simulink model "SLA_1a"  (R2023a)
settings: Solver=ode4  StartTime=0.0  StopTime=20  FixedStep=0.005  RelTol=1e-3
InitFcn:
  | SLA
values from neighbouring files (symbols this model uses):
  K_scheduled = zeros(length(V_op), 2)    [CAL3.m]    (also in CUB.m; DLC2.m; MUS.m; OHZ.m)
  V_op = 5:5:85    [CAL3.m]    (also in CUB.m; DLC2.m; MUS.m; OHZ.m)
  X_track = [linspace(0, runway_length, 200)'; runway_length + R_track * cos(theta_circ(2:end))]    [CAL3.m]    (also in CUB.m = [0; 5000]; DLC2.m = 0:0.1:total_track_length; MUS.m = [0; 2000]; OHZ.m = [0; 2000])
  Y_track = [zeros(200, 1); R_track + R_track * sin(theta_circ(2:end))]    [CAL3.m]    (also in CUB.m = [0; 0]; DLC2.m = zeros(size(X_track)); MUS.m = [0; 0]; OHZ.m = [0; 0])
libraries: simulink x2, slpidlib x1
(part 1 of 2)
settings Model: NumberOfSteps=1000  SnapshotBufferSize=1000  SnapshotInterval=1000  Creator=KBISWAS  LastModifiedBy=KBISWAS

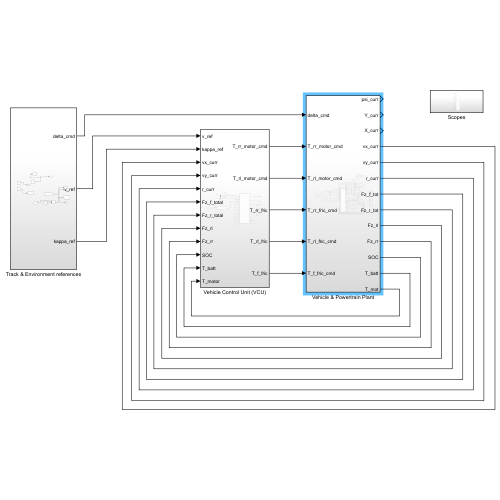
[thumbnail: Simulink's stored preview of the top-level diagram]
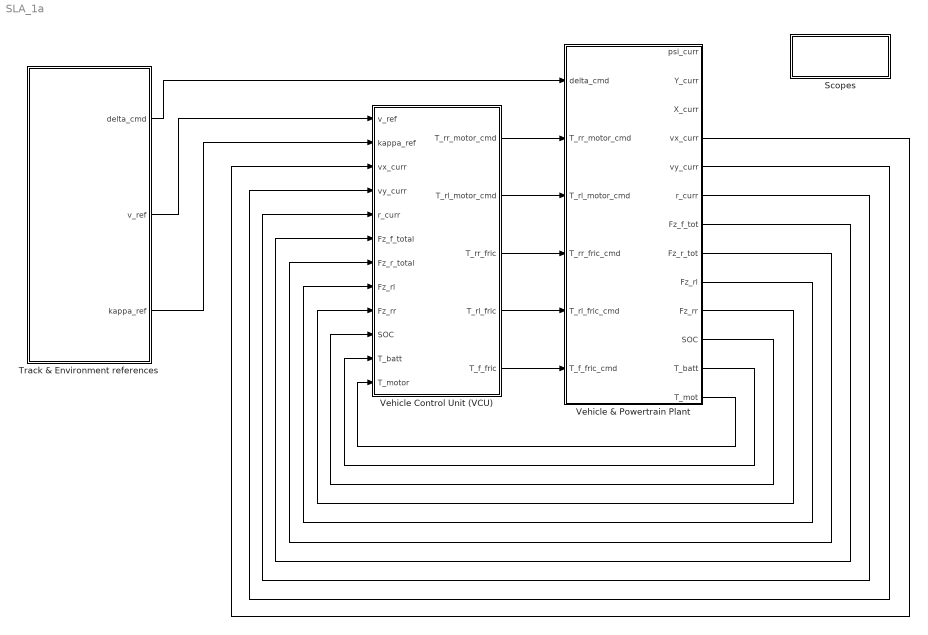
== system SLA_1a ==
  Scopes : Subsystem
  Track & Environment references : Subsystem
  Vehicle & Powertrain Plant : Subsystem
  Vehicle Control Unit (VCU) : Subsystem
  wires:
  Track & Environment references/2(v_ref) -> Vehicle Control Unit (VCU)/1(v_ref)
  Vehicle Control Unit (VCU)/1(T_rr_motor_cmd) -> Vehicle & Powertrain Plant/2(T_rr_motor_cmd)
  Track & Environment references/3(kappa_ref) -> Vehicle Control Unit (VCU)/2(kappa_ref)
  Track & Environment references/1(delta_cmd) -> Vehicle & Powertrain Plant/1(delta_cmd)
  Vehicle Control Unit (VCU)/2(T_rl_motor_cmd) -> Vehicle & Powertrain Plant/3(T_rl_motor_cmd)
  Vehicle Control Unit (VCU)/3(T_rr_fric) -> Vehicle & Powertrain Plant/4(T_rr_fric_cmd)
  Vehicle Control Unit (VCU)/4(T_rl_fric) -> Vehicle & Powertrain Plant/5(T_rl_fric_cmd)
  Vehicle Control Unit (VCU)/5(T_f_fric) -> Vehicle & Powertrain Plant/6(T_f_fric_cmd)
  Vehicle & Powertrain Plant/4(vx_curr) -> Vehicle Control Unit (VCU)/3(vx_curr)
  Vehicle & Powertrain Plant/5(vy_curr) -> Vehicle Control Unit (VCU)/4(vy_curr)
  Vehicle & Powertrain Plant/6(r_curr) -> Vehicle Control Unit (VCU)/5(r_curr)
  Vehicle & Powertrain Plant/7(Fz_f_tot) -> Vehicle Control Unit (VCU)/6(Fz_f_total)
  Vehicle & Powertrain Plant/8(Fz_r_tot) -> Vehicle Control Unit (VCU)/7(Fz_r_total)
  Vehicle & Powertrain Plant/9(Fz_rl) -> Vehicle Control Unit (VCU)/8(Fz_rl)
  Vehicle & Powertrain Plant/10(Fz_rr) -> Vehicle Control Unit (VCU)/9(Fz_rr)
  Vehicle & Powertrain Plant/11(SOC) -> Vehicle Control Unit (VCU)/10(SOC)
  Vehicle & Powertrain Plant/12(T_batt) -> Vehicle Control Unit (VCU)/11(T_batt)
  Vehicle & Powertrain Plant/13(T_mot) -> Vehicle Control Unit (VCU)/12(T_motor)

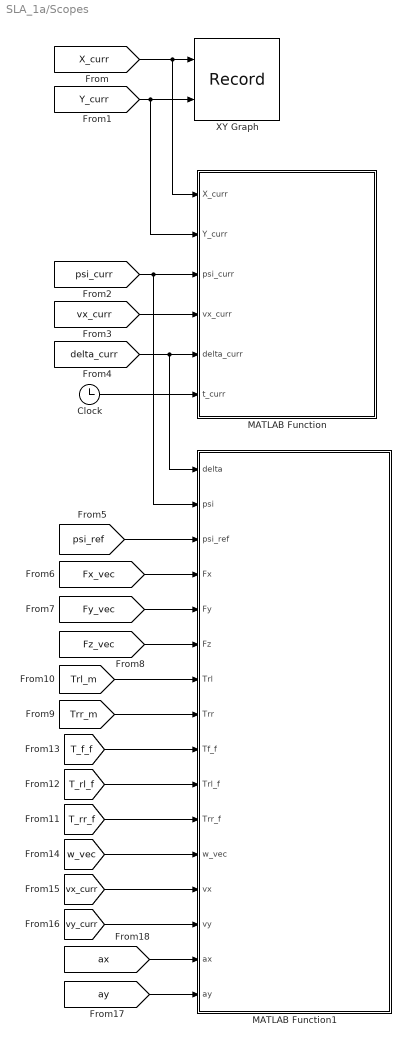
== system SLA_1a/Scopes ==
  Clock : Clock
  MATLAB Function : MATLAB Function  TreatAsAtomicUnit=on
  MATLAB Function1 : MATLAB Function  TreatAsAtomicUnit=on
  XY Graph : Record  FileSettingsInternal="{\"entries\":[{\"content\":{\"excelSettings\":{\"content\":{},\"type\":\"Streamout.ExcelSettings\"}},\"type\":\"Streamout.FileSettingStorage\",\"uuid\":\"\"}],\"packageUris\":[\"http:\\/\\/schema.mathworks.com\\/mf0\\/streamout_blocks\\/R2020a\"],\"version\":\"1.0\"}"  Layout=[1 1]  SignalsInternal="{\"entries\":[{\"content\":{\"signals\":[{\"content\":{\"blockPath\":[],\"dimensions\":[1],\"domain\":\"\",\"lineColor\":\"#a2142f\",\"plots\":[1],\"port\":1,\"signalID\":11566,\"signalName\":\"From\"},\"type\":\"RecordBlkView.Signal\",\"uuid\":\"\"},{\"content\":{\"blockPath\":[],\"dimensions\":[1],\"domain\":\"\",\"lineColor\":\"#139fff\",\"plots\":[1],\"port\":2,\"signalID\":11569,\"signalName\":\"From1\"},\"type\":\"RecordBlkView.Signal\",\"uuid\":\"\"}]},\"type\":\"RecordBlkView.InputSignals\",\"uuid\":\"\"}],\"packageUris\":[\"http:\\/\\/schema.mathworks.com\\/mf0\\/streamout_blocks\\/R2020a\"],\"version\":\"1.0\"}"  VisualizationBindings="{\"xyplotplugin\":{\"info\":[{\"series\":[{\"bindingParametersList\":[{\"parameter\":\"X-Axis\",\"signalID\":11566,\"signalName\":\"From\"},{\"parameter\":\"Y-Axis\",\"signalID\":11569,\"signalName\":\"From1\"}],\"seriesID\":14015}],\"subplotID\":1}]}}"  CompatibilityTag=XY
  wires:
  [X_curr] -> MATLAB Function/1(X_curr), XY Graph/1
  [Y_curr] -> MATLAB Function/2(Y_curr), XY Graph/2
  [psi_curr] -> MATLAB Function/3(psi_curr), MATLAB Function1/2(psi)
  [vx_curr] -> MATLAB Function/4(vx_curr)
  [delta_curr] -> MATLAB Function1/1(delta), MATLAB Function/5(delta_curr)
  Clock/1 -> MATLAB Function/6(t_curr)
  [psi_ref] -> MATLAB Function1/3(psi_ref)
  [Fx_vec] -> MATLAB Function1/4(Fx)
  [Fy_vec] -> MATLAB Function1/5(Fy)
  [Fz_vec] -> MATLAB Function1/6(Fz)
  [Trr_m] -> MATLAB Function1/8(Trr)
  [Trl_m] -> MATLAB Function1/7(Trl)
  [T_f_f] -> MATLAB Function1/9(Tf_f)
  [T_rr_f] -> MATLAB Function1/11(Trr_f)
  [T_rl_f] -> MATLAB Function1/10(Trl_f)
  [w_vec] -> MATLAB Function1/12(w_vec)
  [vx_curr] -> MATLAB Function1/13(vx)
  [vy_curr] -> MATLAB Function1/14(vy)
  [ax] -> MATLAB Function1/15(ax)
  [ay] -> MATLAB Function1/16(ay)

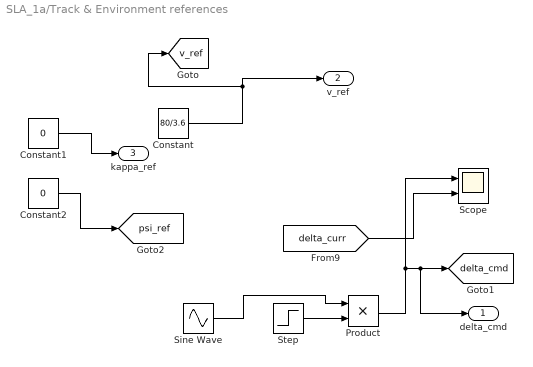
== system SLA_1a/Track & Environment references ==
  Constant : Constant  Value=80/3.6
  Constant1 : Constant  Value=0
  Constant2 : Constant  Value=0
  Product : Product
  Scope : Scope  NumInputPorts=2
  Sine Wave : Sin  Amplitude=0.1  Frequency=4  Phase=0.703  SampleTime=0
  Step : Step  Time=7  SampleTime=0
  delta_cmd : Outport
  v_ref : Outport  Port=2
  kappa_ref : Outport  Port=3
  tag scope: delta_cmd=global, psi_ref=global, v_ref=global
  wires:
  Constant2/1 -> [psi_ref]
  Constant1/1 -> kappa_ref/1
  Constant/1 -> v_ref/1, [v_ref]
  Product/1 -> [delta_cmd], delta_cmd/1, Scope/1
  [delta_curr] -> Scope/2
  Step/1 -> Product/2
  Sine Wave/1 -> Product/1

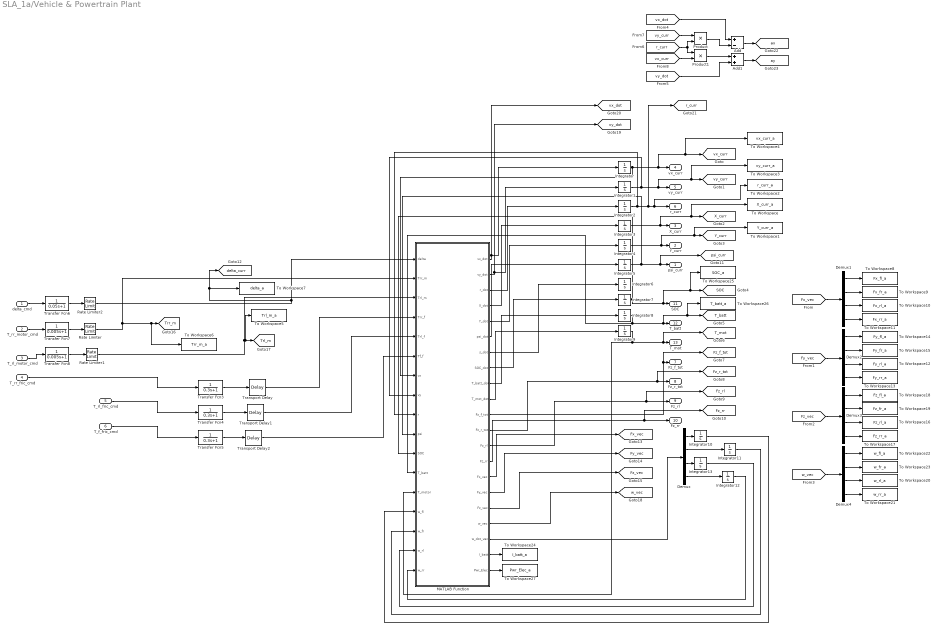
== system SLA_1a/Vehicle & Powertrain Plant ==
  delta_cmd : Inport
  T_rr_motor_cmd : Inport  Port=2
  T_rl_motor_cmd : Inport  Port=3
  T_rr_fric_cmd : Inport  Port=4
  T_rl_fric_cmd : Inport  Port=5
  T_f_fric_cmd : Inport  Port=6
  Add : Sum  Inputs=+-
  Add1 : Sum
  Demux{,1..4} (5 alike) : Demux
  Integrator : Integrator  InitialCondition=5
  Integrator{1..6,10..13} (10 alike) : Integrator
  Integrator7 : Integrator  InitialCondition=0.9
  Integrator8 : Integrator  InitialCondition=30
  Integrator9 : Integrator  InitialCondition=30
  MATLAB Function : MATLAB Function  TreatAsAtomicUnit=on
  Product : Product
  Product1 : Product
  Rate Limiter : RateLimiter  RisingSlewLimit=500  FallingSlewLimit=-500  SampleTimeMode=inherited
  Rate Limiter1 : RateLimiter  RisingSlewLimit=500  FallingSlewLimit=-500  SampleTimeMode=inherited
  Rate Limiter2 : RateLimiter  RisingSlewLimit=10  FallingSlewLimit=-10  SampleTimeMode=inherited
  To Workspace : ToWorkspace  VariableName=X_curr_a  SaveFormat=Timeseries  SampleTime=-1
  To Workspace1 : ToWorkspace  VariableName=Y_curr_a  SaveFormat=Timeseries  SampleTime=-1
  To Workspace10 : ToWorkspace  VariableName=Fx_rl_a  SaveFormat=Timeseries  SampleTime=-1
  To Workspace11 : ToWorkspace  VariableName=Fx_rr_a  SaveFormat=Timeseries  SampleTime=-1
  To Workspace12 : ToWorkspace  VariableName=Fy_rl_a  SaveFormat=Timeseries  SampleTime=-1
  To Workspace13 : ToWorkspace  VariableName=Fy_rr_a  SaveFormat=Timeseries  SampleTime=-1
  To Workspace14 : ToWorkspace  VariableName=Fy_fl_a  SaveFormat=Timeseries  SampleTime=-1
  To Workspace15 : ToWorkspace  VariableName=Fy_fr_a  SaveFormat=Timeseries  SampleTime=-1
  To Workspace16 : ToWorkspace  VariableName=Fz_rl_a  SaveFormat=Timeseries  SampleTime=-1
  To Workspace17 : ToWorkspace  VariableName=Fz_rr_a  SaveFormat=Timeseries  SampleTime=-1
  To Workspace18 : ToWorkspace  VariableName=Fz_fl_a  SaveFormat=Timeseries  SampleTime=-1
  To Workspace19 : ToWorkspace  VariableName=Fz_fr_a  SaveFormat=Timeseries  SampleTime=-1
  To Workspace2 : ToWorkspace  VariableName=r_curr_a  SaveFormat=Timeseries  SampleTime=-1
  To Workspace20 : ToWorkspace  VariableName=w_rl_a  SaveFormat=Timeseries  SampleTime=-1
  To Workspace21 : ToWorkspace  VariableName=w_rr_a  SaveFormat=Timeseries  SampleTime=-1
  To Workspace22 : ToWorkspace  VariableName=w_fl_a  SaveFormat=Timeseries  SampleTime=-1
  To Workspace23 : ToWorkspace  VariableName=w_fr_a  SaveFormat=Timeseries  SampleTime=-1
  To Workspace24 : ToWorkspace  VariableName=I_batt_a  SaveFormat=Timeseries  SampleTime=-1
  To Workspace25 : ToWorkspace  VariableName=SOC_a  SaveFormat=Timeseries  SampleTime=-1
  To Workspace26 : ToWorkspace  VariableName=T_batt_a  SaveFormat=Timeseries  SampleTime=-1
  To Workspace27 : ToWorkspace  VariableName=Pwr_Elec_a  SaveFormat=Timeseries  SampleTime=-1
  To Workspace3 : ToWorkspace  VariableName=vy_curr_a  SaveFormat=Timeseries  SampleTime=-1
  To Workspace4 : ToWorkspace  VariableName=vx_curr_a  SaveFormat=Timeseries  SampleTime=-1
  To Workspace5 : ToWorkspace  VariableName=Trl_m_a  SaveFormat=Timeseries  SampleTime=-1
  To Workspace6 : ToWorkspace  VariableName=Trr_m_a  SaveFormat=Timeseries  SampleTime=-1
  To Workspace7 : ToWorkspace  VariableName=delta_a  SaveFormat=Timeseries  SampleTime=-1
  To Workspace8 : ToWorkspace  VariableName=Fx_fl_a  SaveFormat=Timeseries  SampleTime=-1
  To Workspace9 : ToWorkspace  VariableName=Fx_fr_a  SaveFormat=Timeseries  SampleTime=-1
  Transfer Fcn3 : TransferFcn  Denominator=[0.3 1]
  Transfer Fcn4 : TransferFcn  Denominator=[0.3 1]
  Transfer Fcn5 : TransferFcn  Denominator=[0.3 1]
  Transfer Fcn6 : TransferFcn  Numerator=1  Denominator=[0.05 1]
  Transfer Fcn7 : TransferFcn  Denominator=[0.005 1]
  Transfer Fcn8 : TransferFcn  Denominator=[0.005 1]
  Transport Delay : TransportDelay  DelayTime=0.03
  Transport Delay1 : TransportDelay  DelayTime=0.03
  Transport Delay2 : TransportDelay  DelayTime=0.03
  psi_curr : Outport
  Y_curr : Outport  Port=2
  X_curr : Outport  Port=3
  vx_curr : Outport  Port=4
  vy_curr : Outport  Port=5
  r_curr : Outport  Port=6
  Fz_f_tot : Outport  Port=7
  Fz_r_tot : Outport  Port=8
  Fz_rl : Outport  Port=9
  Fz_rr : Outport  Port=10
  SOC : Outport  Port=11
  T_batt : Outport  Port=12
  T_mot : Outport  Port=13
  tag scope: Fx_vec=global, Fy_vec=global, Fz_f_tot=global, Fz_r_tot=global, Fz_rl=global, Fz_rr=global, Fz_vec=global, SOC=global, T_batt=global, T_mot=global, Trl_m=global, Trr_m=global, X_curr=global, Y_curr=global, ax=global, ay=global, delta_curr=global, psi_curr=global, r_curr=global, vx_curr=global, vx_dot=global, vy_curr=global, vy_dot=global, w_vec=global
  wires:
  delta_cmd/1 -> Transfer Fcn6/1
  T_rr_fric_cmd/1 -> Transfer Fcn3/1
  T_rl_fric_cmd/1 -> Transfer Fcn4/1
  T_f_fric_cmd/1 -> Transfer Fcn5/1
  Transfer Fcn6/1 -> Rate Limiter2/1
  Rate Limiter/1 -> MATLAB Function/2(Trr_m), To Workspace6/1, [Trr_m]
  Rate Limiter1/1 -> MATLAB Function/3(Trl_m), To Workspace5/1, [Trl_m]
  Transfer Fcn3/1 -> Transport Delay/1
  Transfer Fcn4/1 -> Transport Delay1/1
  Transfer Fcn5/1 -> Transport Delay2/1
  MATLAB Function/1(vx_dot) -> [vx_dot], Integrator/1
  MATLAB Function/2(vy_dot) -> [vy_dot], Integrator1/1
  MATLAB Function/3(r_dot) -> Integrator2/1
  MATLAB Function/4(X_dot) -> Integrator3/1
  MATLAB Function/5(Y_dot) -> Integrator4/1
  MATLAB Function/6(psi_dot) -> Integrator5/1
  MATLAB Function/7(s_dot) -> Integrator6/1
  MATLAB Function/8(SOC_dot) -> Integrator7/1
  Integrator/1 -> MATLAB Function/7(vx), To Workspace4/1, [vx_curr], vx_curr/1
  Integrator1/1 -> MATLAB Function/8(vy), To Workspace3/1, [vy_curr], vy_curr/1
  Integrator2/1 -> [r_curr], To Workspace2/1, r_curr/1, MATLAB Function/9(r)
  Integrator5/1 -> MATLAB Function/10(psi), [psi_curr], psi_curr/1
  Integrator8/1 -> MATLAB Function/12(T_batt), To Workspace26/1, [T_batt], T_batt/1
  Integrator9/1 -> MATLAB Function/13(T_motor), [T_mot], T_mot/1
  Integrator4/1 -> To Workspace1/1, [Y_curr], Y_curr/1
  Integrator3/1 -> To Workspace/1, [X_curr], X_curr/1
  MATLAB Function/11(Fz_f_tot) -> [Fz_f_tot], Fz_f_tot/1
  Integrator7/1 -> MATLAB Function/11(SOC), To Workspace25/1, [SOC], SOC/1
  MATLAB Function/14(Fz_rr) -> [Fz_rr], Fz_rr/1
  MATLAB Function/15(Fx_vec) -> [Fx_vec]
  MATLAB Function/17(Fz_vec) -> [Fz_vec]
  MATLAB Function/9(T_batt_dot) -> Integrator8/1
  MATLAB Function/10(T_mot_dot) -> Integrator9/1
  MATLAB Function/12(Fz_r_tot) -> [Fz_r_tot], Fz_r_tot/1
  MATLAB Function/13(Fz_rl) -> [Fz_rl], Fz_rl/1
  MATLAB Function/16(Fy_vec) -> [Fy_vec]
  MATLAB Function/18(w_vec) -> [w_vec]
  Demux/4 -> Integrator12/1
  Demux/3 -> Integrator13/1
  Demux/2 -> Integrator11/1
  Demux/1 -> Integrator10/1
  MATLAB Function/19(w_dot_vec) -> Demux/1
  Integrator10/1 -> MATLAB Function/14(w_fl)
  Integrator11/1 -> MATLAB Function/15(w_fr)
  Integrator12/1 -> MATLAB Function/17(w_rr)
  Integrator13/1 -> MATLAB Function/16(w_rl)
  T_rr_motor_cmd/1 -> Transfer Fcn7/1
  Transfer Fcn7/1 -> Rate Limiter/1
  Transfer Fcn8/1 -> Rate Limiter1/1
  T_rl_motor_cmd/1 -> Transfer Fcn8/1
  [Fx_vec] -> Demux1/1
  Demux1/1 -> To Workspace8/1
  Demux1/2 -> To Workspace9/1
  Demux1/3 -> To Workspace10/1
  Demux1/4 -> To Workspace11/1
  Demux2/2 -> To Workspace15/1
  Demux2/4 -> To Workspace13/1
  Demux2/1 -> To Workspace14/1
  [Fy_vec] -> Demux2/1
  Demux2/3 -> To Workspace12/1
  [Fz_vec] -> Demux3/1
  Demux3/1 -> To Workspace18/1
  Demux3/3 -> To Workspace16/1
  Demux3/4 -> To Workspace17/1
  Demux3/2 -> To Workspace19/1
  Demux4/2 -> To Workspace23/1
  Demux4/4 -> To Workspace21/1
  Demux4/1 -> To Workspace22/1
  Demux4/3 -> To Workspace20/1
  [w_vec] -> Demux4/1
  [vy_curr] -> Product/1
  [r_curr] -> Product1/1, Product/2
  Product/1 -> Add/2
  [vx_dot] -> Add/1
  [vx_curr] -> Product1/2
  Product1/1 -> Add1/1
  [vy_dot] -> Add1/2
  Add/1 -> [ax]
  Add1/1 -> [ay]
  MATLAB Function/20(I_batt) -> To Workspace24/1
  MATLAB Function/21(Pwr_Elec) -> To Workspace27/1
  Rate Limiter2/1 -> MATLAB Function/1(delta), To Workspace7/1, [delta_curr]
  Transport Delay/1 -> MATLAB Function/4(Trr_f)
  Transport Delay1/1 -> MATLAB Function/5(Trl_f)
  Transport Delay2/1 -> MATLAB Function/6(Tf_f)

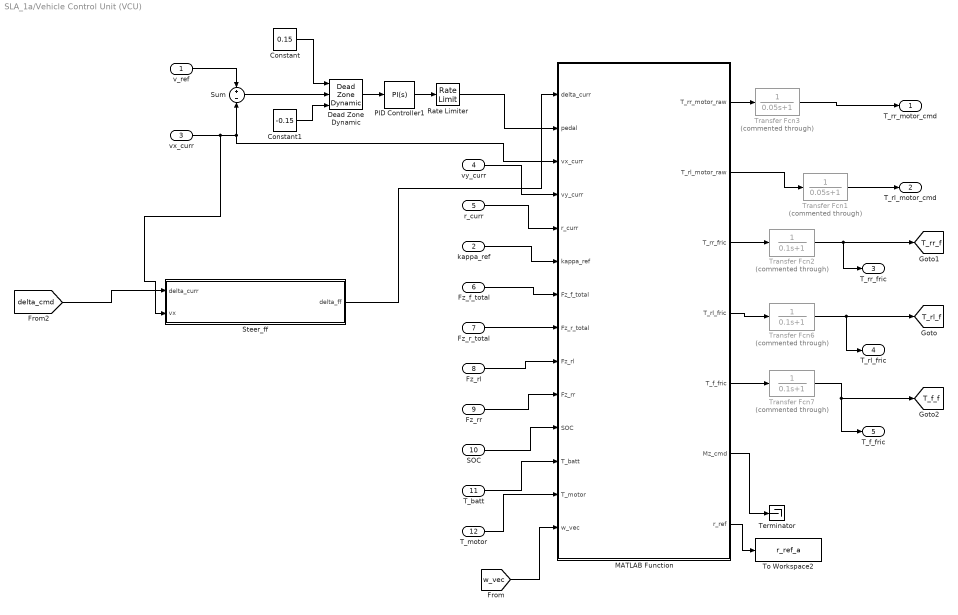
== system SLA_1a/Vehicle Control Unit (VCU) ==
  v_ref : Inport
  kappa_ref : Inport  Port=2
  vx_curr : Inport  Port=3
  vy_curr : Inport  Port=4
  r_curr : Inport  Port=5
  Fz_f_total : Inport  Port=6
  Fz_r_total : Inport  Port=7
  Fz_rl : Inport  Port=8
  Fz_rr : Inport  Port=9
  SOC : Inport  Port=10
  T_batt : Inport  Port=11
  T_motor : Inport  Port=12
  Constant : Constant  Value=0.15
  Constant1 : Constant  Value=-0.15
  Dead Zone Dynamic : simulink/Discontinuities/Dead Zone Dynamic
  MATLAB Function : MATLAB Function  TreatAsAtomicUnit=on
  PID Controller1 : slpidlib/PID Controller  Controller=PI  Form=Parallel  TimeDomain=Continuous-time  UseExternalTs=off  SampleTime=-1  IntegratorMethod=Forward Euler  FilterMethod=Forward Euler  ControllerParametersSource=internal  P=0.2  I=0.1  UseKiTs=off  D=0  N=100  UseFilter=on  TunerSelectOption=Transfer Function Based (PID Tuner App)  InitialConditionSource=internal  InitialConditionForIntegrator=0  InitialConditionForFilter=0  DifferentiatorICPrevScaledInput=0  ExternalReset=none  TrackingMode=off  Kt=1  LimitOutput=on  SatLimitsSource=internal  UpperSaturationLimit=1  LowerSaturationLimit=-1  LinearizeAsGain=on  AntiWindupMode=clamping  Kb=1  LimitIntegrator=off  UpperIntegratorSaturationLimit=inf  LowerIntegratorSaturationLimit=-inf  POutMin=[]  POutMax=[]  IOutMin=[]  IOutMax=[]  DOutMin=[]  DOutMax=[]  NOutMin=[]  NOutMax=[]  SumOutMin=[]  SumOutMax=[]  SaturationOutMin=[]  SaturationOutMax=[]  PParamMin=[]  PParamMax=[]  IParamMin=[]  IParamMax=[]  DParamMin=[]  DParamMax=[]  NParamMin=[]  NParamMax=[]  KbParamMin=[]  KbParamMax=[]  KtParamMin=[]  KtParamMax=[]  KbOutMin=[]  KbOutMax=[]  KtOutMin=[]  KtOutMax=[]  IntegratorOutMin=[]  IntegratorOutMax=[]  FilterOutMin=[]  FilterOutMax=[]  SumI1OutMin=[]  SumI1OutMax=[]  SumI2OutMin=[]  SumI2OutMax=[]  SumI3OutMin=[]  SumI3OutMax=[]  SumI4OutMin=[]  SumI4OutMax=[]  SumDOutMin=[]  SumDOutMax=[]  DifferentiatorOutMin=[]  DifferentiatorOutMax=[]  FilterDiffOutCoefMin=[]  FilterDiffOutCoefMax=[]  ReciprocalOutMin=[]  ReciprocalOutMax=[]  SumDenOutMin=[]  SumDenOutMax=[]  SumNumOutMin=[]  SumNumOutMax=[]  DivideOutMin=[]  DivideOutMax=[]  UdiffTsProdOutMin=[]  UdiffTsProdOutMax=[]  NTsProdOutMin=[]  NTsProdOutMax=[]  UintegralTsProdOutMin=[]  UintegralTsProdOutMax=[]  UngainTsProdOutMin=[]  UngainTsProdOutMax=[]  ClampingZeroOutDataTypeStr=Inherit: Inherit via back propagation  ClampingZeroOutMin=[]  ClampingZeroOutMax=[]  FilterDenConstantOutDataTypeStr=Inherit: Inherit via back propagation  FilterDenConstantOutMin=[]  FilterDenConstantOutMax=[]  PCopyOutDataTypeStr=Inherit: Inherit via back propagation  PCopyOutMin=[]  PCopyOutMax=[]  NCopyOutDataTypeStr=Inherit: Inherit via back propagation  NCopyOutMin=[]  NCopyOutMax=[]  IntegratorContinuousStateAttributes=''  IntegratorStateMustResolveToSignalObject=off  IntegratorRTWStateStorageClass=Auto  FilterContinuousStateAttributes=''  FilterStateMustResolveToSignalObject=off  FilterRTWStateStorageClass=Auto  ParallelPVariant=InternalParameters  IdealPVariant=Disabled  IVariant=InternalParameters  DVariant=Disabled  IntegratorVariant=Continuous  SatVariant=Enabled  AWVariant=ContClampingParallel  PCopyVariant=Disabled  TRVariant=Disabled  FdbkBlocksVariant=Forward  IdealPFdbkVariant=Disabled  SatFdbkVariant=Disabled  DerivativeFilterVariant=Disabled  NVariant=Disabled  NCopyVariant=Disabled_SignalSpec  FilterICVariant=Disabled  IntegratorICVariant=InternalICs  ExternalResetVariant=Disabled  TRSumVariant=Passthrough  SumFdbkVariant=Disabled  SumVariant=Sum_PI  TsampFilterVariant=InternalTs  TsampNgainVariant=Passthrough  TsampIntegralVariant=Disabled_SignalSpec  ExternalSaturationOutDataTypeStr=Inherit: Same as second input
  Rate Limiter : RateLimiter  RisingSlewLimit=2  FallingSlewLimit=-4  SampleTimeMode=inherited
  Steer_ff : Subsystem
  Sum : Sum  Inputs=+-
  Terminator : Terminator
  To Workspace2 : ToWorkspace  VariableName=r_ref_a  SaveFormat=Timeseries  SampleTime=-1
  Transfer Fcn1 : TransferFcn  Commented=through  Denominator=[0.05 1]
  Transfer Fcn2 : TransferFcn  Commented=through  Denominator=[0.1 1]
  Transfer Fcn3 : TransferFcn  Commented=through  Denominator=[0.05 1]
  Transfer Fcn6 : TransferFcn  Commented=through  Denominator=[0.1 1]
  Transfer Fcn7 : TransferFcn  Commented=through  Denominator=[0.1 1]
  T_rr_motor_cmd : Outport
  T_rl_motor_cmd : Outport  Port=2
  T_rr_fric : Outport  Port=3
  T_rl_fric : Outport  Port=4
  T_f_fric : Outport  Port=5
  tag scope: T_f_f=global, T_rl_f=global, T_rr_f=global
  wires:
  v_ref/1 -> Sum/1
  vy_curr/1 -> MATLAB Function/4(vy_curr)
  r_curr/1 -> MATLAB Function/5(r_curr)
  kappa_ref/1 -> MATLAB Function/6(kappa_ref)
  Fz_f_total/1 -> MATLAB Function/7(Fz_f_total)
  Fz_r_total/1 -> MATLAB Function/8(Fz_r_total)
  Fz_rl/1 -> MATLAB Function/9(Fz_rl)
  Fz_rr/1 -> MATLAB Function/10(Fz_rr)
  SOC/1 -> MATLAB Function/11(SOC)
  T_batt/1 -> MATLAB Function/12(T_batt)
  T_motor/1 -> MATLAB Function/13(T_motor)
  Rate Limiter/1 -> MATLAB Function/2(pedal)
  MATLAB Function/1(T_rr_motor_raw) -> Transfer Fcn3/1
  MATLAB Function/2(T_rl_motor_raw) -> Transfer Fcn1/1
  MATLAB Function/3(T_rr_fric) -> Transfer Fcn2/1
  MATLAB Function/4(T_rl_fric) -> Transfer Fcn6/1
  MATLAB Function/5(T_f_fric) -> Transfer Fcn7/1
  MATLAB Function/6(Mz_cmd) -> Terminator/1
  [w_vec] -> MATLAB Function/14(w_vec)
  MATLAB Function/7(r_ref) -> To Workspace2/1
  Steer_ff/1(delta_ff) -> MATLAB Function/1(delta_curr)
  [delta_cmd] -> Steer_ff/1(delta_curr)
  Transfer Fcn3/1 -> T_rr_motor_cmd/1
  Transfer Fcn1/1 -> T_rl_motor_cmd/1
  Transfer Fcn2/1 -> T_rr_fric/1, [T_rr_f]
  Transfer Fcn6/1 -> T_rl_fric/1, [T_rl_f]
  Transfer Fcn7/1 -> T_f_fric/1, [T_f_f]
  Dead Zone Dynamic/1 -> PID Controller1/1
  Constant/1 -> Dead Zone Dynamic/1
  Sum/1 -> Dead Zone Dynamic/2
  PID Controller1/1 -> Rate Limiter/1
  Constant1/1 -> Dead Zone Dynamic/3
  vx_curr/1 -> Steer_ff/2(vx), MATLAB Function/3(vx_curr), Sum/2

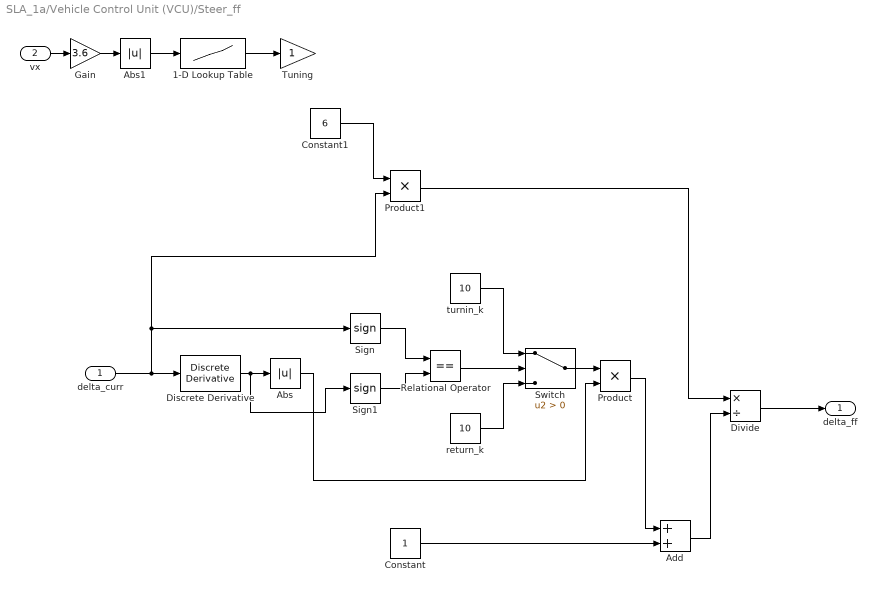
== system SLA_1a/Vehicle Control Unit (VCU)/Steer_ff ==
  delta_curr : Inport
  vx : Inport  Port=2
  1-D Lookup Table : Lookup_n-D  NumberOfTableDimensions=1  LookupTableObject=''  BreakpointsForDimension1=[0 20 40 60 80 100 120 140 160 180 200]  BreakpointsForDimension1FirstPoint=10  BreakpointsForDimension2FirstPoint=10  BreakpointsForDimension1Spacing=12  BreakpointsForDimension2Spacing=12  IndexSearchMethod=Evenly spaced points  Table=[0 2 3.5 3.5 3.5 3.5 3.5 3.5 3 2.5 2]  InterpMethod=Akima spline  DiagnosticForOutOfRangeInput=Error  InternalRulePriority=Speed  RndMeth=Simplest
  Abs : Abs  SaturateOnIntegerOverflow=off
  Abs1 : Abs  SaturateOnIntegerOverflow=off
  Add : Sum
  Constant : Constant
  Constant1 : Constant  Value=6
  Discrete Derivative : simulink/Discrete/Discrete Derivative  gainval=1.0  ICPrevScaledInput=0.0  OutMin=[]  OutMax=[]  OutDataType=fixdt(1, 16)  OutScaling=2^-10  DoSatur=off
  Divide : Product  Inputs=*/
  Gain : Gain  Gain=3.6
  Product : Product
  Product1 : Product
  Relational Operator : RelationalOperator  Operator===  OutDataTypeStr=boolean  RndMeth=Simplest  InputSameDT=off
  Sign : Signum
  Sign1 : Signum
  Switch : Switch  Criteria=u2 > Threshold  SaturateOnIntegerOverflow=off  InputSameDT=off
  Tuning : Gain
  return_k : Constant  Value=10
  turnin_k : Constant  Value=10
  delta_ff : Outport
  wires:
  Product1/1 -> Divide/1
  return_k/1 -> Switch/3
  Switch/1 -> Product/1
  Product/1 -> Add/1
  Sign/1 -> Relational Operator/1
  delta_curr/1 -> Discrete Derivative/1, Product1/2, Sign/1
  Relational Operator/1 -> Switch/2
  Add/1 -> Divide/2
  Discrete Derivative/1 -> Sign1/1, Abs/1
  Abs/1 -> Product/2
  Constant/1 -> Add/2
  Sign1/1 -> Relational Operator/2
  Divide/1 -> delta_ff/1
  turnin_k/1 -> Switch/1
  vx/1 -> Gain/1
  1-D Lookup Table/1 -> Tuning/1
  Gain/1 -> Abs1/1
  Constant1/1 -> Product1/1
  Abs1/1 -> 1-D Lookup Table/1

== matlab function SLA_1a/Scopes/MATLAB Function ==
  settings: updateMethod=DISCRETE
  data: X_curr input; Y_curr input; psi_curr input; vx_curr input; delta_curr input; t_curr input; X_track parameter; Y_track parameter
function live_track_plotter(X_curr, Y_curr, psi_curr, vx_curr, delta_curr, t_curr, X_track, Y_track)
    coder.extrinsic('figure', 'plot', 'hold', 'axis', 'title', 'xlabel', 'ylabel', 'set', 'drawnow', 'animatedline', 'addpoints', 'legend', 'grid', 'patch', 'text');
    
    persistent hFig hCar hTrail hText counter 
    
    if isempty(counter)
        counter = 0;
        
        hFig = figure('Name', 'Circular acceleration tracking', 'Color', 'w', 'Position', [100, 100, 800, 600]);
        plot(X_track, Y_track, '--', 'Color', [0.4 0.4 0.4], 'LineWidth', 1.5); hold on;
        
        plot(X_track(1), Y_track(1), 'ko', 'MarkerSize', 10, 'MarkerFaceColor', 'g', 'LineWidth', 1.5);
        text(X_track(1) - 50, Y_track(1) + 70, 'Start / Finish', 'FontSize', 10, 'FontWeight', 'bold', 'Color', 'k', 'BackgroundColor', [1 1 1 0.7]);
        
        hTrail = animatedline('Color', 'b', 'LineWidth', 1.5);
        
        hCar = patch(0, 0, [0.8 0 0], 'EdgeColor', 'k', 'LineWidth', 1);
        set(hCar, 'FaceAlpha', 0.8); 
        
        hText = text(0, 0, ' Init...', 'FontSize', 10, 'FontWeight', 'bold', 'BackgroundColor', [1 1 1 0.8], 'EdgeColor', 'k', 'Margin', 2);
        
        axis equal; grid on;
        title('Live Vehicle Tracking with Telemetry');
        xlabel('X Position (meters)'); ylabel('Y Position (meters)');
        legend('Reference Track', 'Start/Finish', 'Driven Path', 'EV Position & Heading', 'Telemetry', 'Location', 'best');
    end
    counter = counter + 1;
    
    if mod(counter, 10) == 0
        addpoints(hTrail, X_curr, Y_curr);
        
        % --- REALISTIC 1:1 VEHICLE SCALING ---
        L_vis = 4.5; % 4.5 meters long
        W_vis = 1.9; % 1.9 meters wide
        % ------------------------------------
        
        base_X = [L_vis/2,  L_vis*0.3,   0,       -L_vis*0.35, -L_vis/2,  -L_vis/2,   -L_vis*0.35,  0,        L_vis*0.3,   L_vis/2];
        base_Y = [0,        W_vis*0.45, W_vis/2,  W_vis/2,     W_vis*0.3, -W_vis*0.3, -W_vis/2,    -W_vis/2, -W_vis*0.45, 0];
        
        R = [cos(psi_curr), -sin(psi_curr); 
             sin(psi_curr),  cos(psi_curr)];
             
        rotated_coords = R * [base_X; base_Y];
        final_X = rotated_coords(1, :) + X_curr;
        final_Y = rotated_coords(2, :) + Y_curr;
        
        set(hCar, 'XData', final_X, 'YData', final_Y);
        
        speed_kmh = vx_curr * 3.6;
        steer_deg = delta_curr * (180 / pi);
        
        telemetry_str = sprintf(' Spd: %.1f km/h\n Steer. Ang.: %.1f deg', speed_kmh, steer_deg);
        
        % Brought the text box much closer to the scaled vehicle
        set(hText, 'Position', [X_curr + 10, Y_curr + 10], 'String', telemetry_str);
        
        drawnow limitrate; 
    end
end

== matlab function SLA_1a/Scopes/MATLAB Function1 ==
  settings: updateMethod=DISCRETE
  data: delta input; psi input; psi_ref input; Fx input; Fy input; Fz input; Trl input; Trr input; Tf_f input; Trl_f input; Trr_f input; w_vec input; vx input; vy input; ax input; ay input
function vehicle_frame_plotter(delta, psi, psi_ref, Fx, Fy, Fz, Trl, Trr, Tf_f, Trl_f, Trr_f, w_vec, vx, vy, ax, ay)
    coder.extrinsic('figure', 'plot', 'hold', 'axis', 'title', 'set', 'drawnow', 'patch', 'text', 'line', 'quiver', 'sprintf');
    
    persistent hWheels hSteer hSpokes hPsiRef hPsiAct hFlags hTqFlags hMotors hAxleFront hCircles hGdots hSwLabel hRwLabel hAngleLabel hVelArrow hAccArrow hVelText hAccText hCrosshairs counter
    
    if isempty(counter)
        % =====================================================================
        % STRICT CODER INITIALIZATION
        % =====================================================================
        counter = 0;
        hSteer = 0.0; hPsiRef = 0.0; hPsiAct = 0.0; hAxleFront = 0.0;
        hWheels = zeros(1,4); hFlags = zeros(1,4); hTqFlags = zeros(1,2); hMotors = zeros(1,2);
        hSpokes = zeros(1,3); hCircles = zeros(1,4); hGdots = zeros(1,4);
        hSwLabel = 0.0; hRwLabel = 0.0; hAngleLabel = 0.0;
        hVelArrow = 0.0; hAccArrow = 0.0; hVelText = 0.0; hAccText = 0.0;
        hCrosshairs = zeros(1,2);
        
        figure('Name', 'Vehicle Frame Telemetry - Car A', 'Color', 'w', 'Position', [100, 100, 750, 750]);
        hold on;
        
        % Chassis Outline & Front Axle
        plot([-1, 1, 1, -1, -1], [2, 2, -2, -2, 2], 'k', 'LineWidth', 2);
        hAxleFront = double(line([1, -1], [1.5, 1.5], 'Color', [0.2 0.2 0.2], 'LineWidth', 2));
        
        % Wheels Array Setup [FL, FR, RL, RR]
        for i = 1:4; hWheels(i) = double(patch(0, 0, [0.3 0.3 0.3])); end
        
        % =====================================================================
        % FRICTION CIRCLES, STEERING WHEEL, & YAW VECTORS
        % =====================================================================
        th_c = 0:0.1:2*pi;
        circle_x = cos(th_c); circle_y = sin(th_c);
        c_pos = [-2.0, 2.3; 2.0, 2.3; -2.0, -2.3; 2.0, -2.3]; 
        for i = 1:4
            hCircles(i) = double(plot(c_pos(i,1) + 0.5*circle_x, c_pos(i,2) + 0.5*circle_y, 'Color', [0.6 0 0.6], 'LineStyle', '--', 'LineWidth', 1.2));
            hGdots(i) = double(plot(c_pos(i,1), c_pos(i,2), 'mo', 'MarkerFaceColor', 'm', 'MarkerSize', 5));
        end
        
        hSteer = double(plot(0.4*cos(th_c), 0.4*sin(th_c) + 0.5, 'k', 'LineWidth', 3));
        hSpokes(1) = double(line([0, 0], [0.5, 0.5], 'Color', 'k', 'LineWidth', 2.5));
        hSpokes(2) = double(line([0, 0], [0.5, 0.5], 'Color', 'k', 'LineWidth', 2.5));
        hSpokes(3) = double(line([0, 0], [0.5, 0.5], 'Color', 'k', 'LineWidth', 2.5));
        
        hPsiRef = double(quiver(0, 1.8, 0, 0.8, 'r', 'LineWidth', 2.5, 'MaxHeadSize', 2));
        hPsiAct = double(quiver(0, 1.8, 0, 0.8, 'b', 'LineWidth', 2.5, 'MaxHeadSize', 2));
        
        for i = 1:4; hFlags(i) = double(text(0, 0, '', 'FontSize', 8, 'BackgroundColor', [1 1 1 0.8], 'EdgeColor', 'k')); end
        
        % =====================================================================
        % VEHICLE A POWERTRAIN GRAPHIC (Dual Motors)
        % =====================================================================
        m_b = [-.15, .15, .15, -.15]; m_w = [.2, .2, -.2, -.2];
        hMotors(1) = double(patch(m_b - 0.6, m_w - 1.5, [0.5 0.5 0.5])); % Left Motor
        hMotors(2) = double(patch(m_b + 0.6, m_w - 1.5, [0.5 0.5 0.5])); % Right Motor
        
        hTqFlags(1) = double(text(-0.6, -0.9, '', 'FontSize', 10, 'FontWeight', 'bold', 'HorizontalAlignment', 'center'));
        hTqFlags(2) = double(text(0.6, -0.9, '', 'FontSize', 10, 'FontWeight', 'bold', 'HorizontalAlignment', 'center'));
        
        % Labels
        hSwLabel = double(text(0, 1.2, '', 'FontSize', 9, 'FontWeight', 'bold', 'HorizontalAlignment', 'center'));
        hRwLabel = double(text(0, 1.65, '', 'FontSize', 9, 'FontWeight', 'bold', 'HorizontalAlignment', 'center', 'Color', [0 0.5 0]));
        hAngleLabel = double(text(0, 2.8, '', 'FontSize', 10, 'FontWeight', 'bold', 'HorizontalAlignment', 'center', 'Color', [0.4 0 0.6]));

        % =====================================================================
        % SHARED-ORIGIN VELOCITY & ACCELERATION VECTORS
        % =====================================================================
        hCrosshairs(1) = double(plot([-2.0 2.0], [-3.8 -3.8], 'k:', 'Color', [0.7 0.7 0.7]));
        hCrosshairs(2) = double(plot([0 0], [-4.2 -1.8], 'k:', 'Color', [0.7 0.7 0.7]));

        hVelArrow = double(quiver(0, -3.8, 0, 0, 'Color', [0 0.4 0.8], 'LineWidth', 2.5, 'MaxHeadSize', 2, 'AutoScale', 'off'));
        hAccArrow = double(quiver(0, -3.8, 0, 0, 'Color', [0.8 0.3 0], 'LineWidth', 2.5, 'MaxHeadSize', 2, 'AutoScale', 'off'));

        hVelText = double(text(-2.0, -4.3, '', 'FontSize', 9, 'FontWeight', 'bold', 'HorizontalAlignment', 'center', 'Color', [0 0.4 0.8]));
        hAccText = double(text(2.0, -4.3, '', 'FontSize', 9, 'FontWeight', 'bold', 'HorizontalAlignment', 'center', 'Color', [0.8 0.3 0]));
        
        axis([-4.5 4.5 -4.5 4.5]); axis equal; grid on;
        title('Dynamics - Car A (Dual Motor): Forces & Friction Circles');
    end
    counter = counter + 1;
    
    % --- UPDATE LOOP ---
    if mod(counter, 10) == 0
        R_delta = [cos(delta) -sin(delta); sin(delta) cos(delta)];
        w_orig = [-.2 .2 .2 -.2; .4 .4 -.4 -.4]; 
        w_rot = R_delta * w_orig;
        
        set(hWheels(1), 'XData', w_rot(1,:) - 1, 'YData', w_rot(2,:) + 1.5); 
        set(hWheels(2), 'XData', w_rot(1,:) + 1, 'YData', w_rot(2,:) + 1.5); 
        set(hWheels(3), 'XData', w_orig(1,:) - 1, 'YData', w_orig(2,:) - 1.5); 
        set(hWheels(4), 'XData', w_orig(1,:) + 1, 'YData', w_orig(2,:) - 1.5); 
        
        set(hAxleFront, 'XData', [mean(w_rot(1,:) - 1), mean(w_rot(1,:) + 1)], 'YData', [mean(w_rot(2,:) + 1.5), mean(w_rot(2,:) + 1.5)]);
        
        sw_a = delta * 14; 
        th_sw = (0:0.1:2*pi) + sw_a;
        set(hSteer, 'XData', 0.4*cos(th_sw), 'YData', 0.4*sin(th_sw) + 0.5);
        spk = [0, pi, 1.5*pi] + sw_a;
        for j=1:3; set(hSpokes(j), 'XData', [0, 0.4*cos(spk(j))], 'YData', [0.5, 0.5 + 0.4*sin(spk(j))]); end
        
        set(hSwLabel, 'String', sprintf('SW: %.1f deg', sw_a * 180/pi));
        set(hRwLabel, 'String', sprintf('RW: %.1f deg', delta * 180/pi));
        
        psi_e = psi_ref - psi; 
        set(hPsiRef, 'UData', 0.8*sin(psi_e), 'VData', 0.8*cos(psi_e));
        set(hPsiAct, 'UData', 0, 'VData', 0.8);
        set(hAngleLabel, 'String', sprintf('Sideslip: %.1f deg', psi_e * 180/pi));
        
        fb = [abs(Tf_f/2), abs(Tf_f/2), abs(Trl_f), abs(Trr_f)]; 
        mu = 1.0;
        c_pos = [-2.0, 2.3; 2.0, 2.3; -2.0, -2.3; 2.0, -2.3]; 
        th_c = 0:0.1:2*pi;
        rpm_vec = w_vec * (30 / pi);
        
        for i = 1:4
            if fb(i) > 5; set(hWheels(i), 'FaceColor', [0.8 0 0]); else set(hWheels(i), 'FaceColor', [0.3 0.3 0.3]); end
            F_max = max(100, mu * Fz(i));
            scale = 0.5 / 6000; 
            set(hCircles(i), 'XData', c_pos(i,1) + F_max*scale*cos(th_c), 'YData', c_pos(i,2) + F_max*scale*sin(th_c));
            set(hGdots(i), 'XData', c_pos(i,1) + Fy(i)*scale, 'YData', c_pos(i,2) + Fx(i)*scale);
        end
        
        % Dual Motor Visualization Logic
        mt = [Trl, Trr]; 
        for k = 1:2
            if mt(k) > 0.1; set(hMotors(k), 'FaceColor', [0 0.7 0]); 
            elseif mt(k) < -0.1; set(hMotors(k), 'FaceColor', [0.7 0 0]); 
            else set(hMotors(k), 'FaceColor', [0.5 0.5 0.5]); end
            
            set(hTqFlags(k), 'String', sprintf('%.1f Nm', mt(k)));
        end
        
        pos = [-4.1, 1.5; 2.8, 1.5; -4.1, -1.5; 2.8, -1.5]; 
        for i = 1:4
            f_str = sprintf('Fx: %.0f\nFy: %.0f\nFz: %.0f\nFric: %.1f\nRPM: %.0f', Fx(i), Fy(i), Fz(i), fb(i), rpm_vec(i));
            set(hFlags(i), 'Position', [pos(i,1), pos(i,2)], 'String', f_str);
        end

        % =====================================================================
        % UPDATE DYNAMIC VECTORS
        % =====================================================================
        vx_kmh = vx * 3.6;
        vy_kmh = vy * 3.6;
        ax_g = ax / 9.81;
        ay_g = ay / 9.81;

        vel_scale = 0.015; 
        acc_scale = 0.8;   

        set(hVelArrow, 'UData', -vy_kmh * vel_scale, 'VData', vx_kmh * vel_scale);
        set(hAccArrow, 'UData', -ay_g * acc_scale, 'VData', ax_g * acc_scale);

        set(hVelText, 'String', sprintf('Vx: %.1f | Vy: %.1f\n[km/h]', vx_kmh, vy_kmh));
        set(hAccText, 'String', sprintf('Ax: %.2f | Ay: %.2f\n[G]', ax_g, ay_g));
        
        drawnow limitrate;
    end
end

== matlab function SLA_1a/Vehicle Control Unit (VCU)/MATLAB Function ==
  settings: updateMethod=DISCRETE
  data: delta_curr input; pedal input; T_rr_motor_raw output; vx_curr input; vy_curr input; r_curr input; kappa_ref input; Fz_f_total input; Fz_r_total input; Fz_rl input; Fz_rr input; SOC input; T_batt input; T_motor input; V_op parameter; K_scheduled parameter; T_rl_motor_raw output; T_rr_fric output; w_vec input; T_rl_fric output; T_f_fric output; Mz_cmd output; r_ref output
function [T_rr_motor_raw, T_rl_motor_raw, T_rr_fric, T_rl_fric, T_f_fric, Mz_cmd, r_ref] = vcu_allocator(delta_curr, pedal, vx_curr, vy_curr, r_curr, kappa_ref, Fz_f_total, Fz_r_total, Fz_rl, Fz_rr, SOC, T_batt, T_motor, V_op, K_scheduled, w_vec)
T_rr_motor_raw = 0.0;
T_rl_motor_raw = 0.0;
T_rr_fric = 0.0;
T_rl_fric = 0.0;
T_f_fric = 0.0;
Mz_cmd = 0.0;

Rw = 0.34; tw = 1.65; G = 10; mu_max = 1.2;

% --- Per-Motor Limits (Total System = 500 kW, 800 Nm) ---
P_motor_base = 250000; % 250 kW per motor
T_motor_max = 400;     % 400 Nm per motor
T_fric_max_per_wheel = 3500;
% --------------------------------------------------------

% --- Battery and Thermal Derating ---
T_batt_cal = [-10, 0, 15, 45, 55, 60]; P_derate_batt_cal = [0, 0.5, 1.0, 1.0, 0.2, 0];
T_motor_cal = [30, 90, 110, 130, 150]; P_derate_motor_cal = [1.0, 1.0, 0.8, 0.2, 0];
SOC_vec = [0, 0.05, 0.15, 0.85, 0.95, 1.0];
P_derate_SOC_dis = [0, 0.1, 1.0, 1.0, 1.0, 1.0]; P_derate_SOC_chg = [1.0, 1.0, 1.0, 1.0, 0.1, 0];

derate_T_batt = interp1(T_batt_cal, P_derate_batt_cal, T_batt(1), 'linear', 0);
derate_T_mot = interp1(T_motor_cal, P_derate_motor_cal, T_motor(1), 'linear', 0);
derate_T_total = min(derate_T_batt, derate_T_mot);

derate_S_dis = interp1(SOC_vec, P_derate_SOC_dis, SOC(1), 'linear', 0);
derate_S_chg = interp1(SOC_vec, P_derate_SOC_chg, SOC(1), 'linear', 0);

P_avail_dis = P_motor_base * min(derate_T_total, derate_S_dis);
P_avail_chg = P_motor_base * min(derate_T_total, derate_S_chg);

vx_lqr = max(vx_curr(1), 5.0);

% --- Speed-based Torque Vectoring Blending (45 km/h to 50 km/h) ---
vx_kmh = vx_curr(1) * 3.6;
tv_blend_lower = 45.0;
tv_blend_upper = 50.0;
if vx_kmh >= tv_blend_upper
    tv_blend = 1.0;
elseif vx_kmh <= tv_blend_lower
    tv_blend = 0.0;
else
    tv_blend = (vx_kmh - tv_blend_lower) / (tv_blend_upper - tv_blend_lower);
end

% --- LQR Yaw Moment Calculation ---
K_dyn_1 = interp1(V_op, K_scheduled(:,1), vx_lqr, 'linear', 'extrap');
K_dyn_2 = interp1(V_op, K_scheduled(:,2), vx_lqr, 'linear', 'extrap');

% =========================================================================
% 1. DYNAMIC ACKERMANN REFERENCE
% =========================================================================
L = 2.6;            % Wheelbase
K_us = 0.0015;      % Small understeer gradient (optional)
r_ref_raw = (vx_lqr * delta_curr(1)) / (L * (1 + K_us * vx_lqr^2));

% =========================================================================
% 2. PHYSICAL YAW RATE BOUNDING (The Jitter Fix)
% =========================================================================
g = 9.81;
% Calculate the absolute maximum yaw rate the tires can sustain
% based on current speed and track friction (r_max = mu * g / Vx)
% We use 0.95 as a safety margin to prevent fighting the TCS limiters.
r_max_phys = (mu_max * g * 0.95) / vx_lqr;

% Clamp the reference so the LQR never demands an impossible turn
r_ref = max(-r_max_phys, min(r_max_phys, r_ref_raw));

% =========================================================================
TV_Bite_Factor = 1;
vy_factor = 1;
Mz_req = tv_blend * -(vy_factor * K_dyn_1(1) * vy_curr(1) + TV_Bite_Factor * K_dyn_2(1) * (r_curr(1) - r_ref));

Mz_cmd = max(-2500, min(2500, Mz_req));
T_delta_wheel_raw = max(-1500, min(1500, (Mz_cmd * Rw) / tw));

% =========================================================================
% --- DYNAMIC MOTOR POWER LIMITS (Hyperbolic Torque Derating) ---
% =========================================================================
% Calculate actual motor speed from wheel speed (rad/s)
% w_vec = [w_fl, w_fr, w_rl, w_rr]
w_motor_rl = max(abs(w_vec(3) * G), 0.1); % Prevent div-by-zero at standstill
w_motor_rr = max(abs(w_vec(4) * G), 0.1);

% Power-limited torque curve: T_max = P_max / w
T_limit_rl_dis = P_avail_dis / w_motor_rl;
T_limit_rr_dis = P_avail_dis / w_motor_rr;
T_limit_rl_chg = P_avail_chg / w_motor_rl;
T_limit_rr_chg = P_avail_chg / w_motor_rr;

% Final motor bounds (Minimum of Inverter current limit and Power limit)
T_motor_lim_rl_dis = min(T_motor_max, T_limit_rl_dis);
T_motor_lim_rr_dis = min(T_motor_max, T_limit_rr_dis);
T_motor_lim_rl_chg = max(-T_motor_max, -T_limit_rl_chg);
T_motor_lim_rr_chg = max(-T_motor_max, -T_limit_rr_chg);

% =========================================================================
T_grip_lim_rl_wheel = mu_max * Fz_rl(1) * Rw * 0.90;
T_grip_lim_rr_wheel = mu_max * Fz_rr(1) * Rw * 0.90;

% Combine physical motor limits with dynamic grip limits
T_max_rl_motor = min(T_motor_lim_rl_dis, T_grip_lim_rl_wheel / G);
T_max_rr_motor = min(T_motor_lim_rr_dis, T_grip_lim_rr_wheel / G);
T_min_rl_motor = max(T_motor_lim_rl_chg, -T_grip_lim_rl_wheel / G);
T_min_rr_motor = max(T_motor_lim_rr_chg, -T_grip_lim_rr_wheel / G);

weight_rl = Fz_rl(1) / max(1, (Fz_rl(1) + Fz_rr(1)));
weight_rr = Fz_rr(1) / max(1, (Fz_rl(1) + Fz_rr(1)));

% --- DRIVE MODE ---
if pedal(1) >= 0
    % Total requested drive torque, limited by combined max capabilities
    T_req_total_motor = pedal(1) * (T_max_rl_motor + T_max_rr_motor);
    T_rr_base_motor = T_req_total_motor * weight_rr;
    T_rl_base_motor = T_req_total_motor * weight_rl;
    
    T_rr_ideal = max(T_min_rr_motor, min(T_max_rr_motor, T_rr_base_motor + (T_delta_wheel_raw/G)));
    T_rl_ideal = max(T_min_rl_motor, min(T_max_rl_motor, T_rl_base_motor - (T_delta_wheel_raw/G)));
    
    % Traction Control (TCS) - Virtual Differential Logic Update
    v_hub_rl = max(vx_curr(1) - (tw/2)*r_curr(1), 1.0);
    v_hub_rr = max(vx_curr(1) + (tw/2)*r_curr(1), 1.0);
    
    kappa_rl = (w_vec(3)*Rw - v_hub_rl) / v_hub_rl;
    kappa_rr = (w_vec(4)*Rw - v_hub_rr) / v_hub_rr;
    
    slip_target = 0.10;
    Kp_tcs = 1000;
    
    % NEW LOGIC: Find the worst-case slip across the axle
    worst_kappa_rear = max(kappa_rl, kappa_rr);
    
    if worst_kappa_rear > slip_target
        % Calculate a single, unified torque penalty
        T_tcs_penalty = Kp_tcs * (worst_kappa_rear - slip_target);
        
        % Apply the EXACT same penalty to BOTH motors. 
        % This links them together and kills asymmetric thrust during a single-wheel slip.
        T_rl_ideal = max(0, T_rl_ideal - T_tcs_penalty);
        T_rr_ideal = max(0, T_rr_ideal - T_tcs_penalty);
    end
    
    T_rr_fric = 0; T_rl_fric = 0; T_f_fric = 0;

% --- BRAKE MODE ---
else
    bias_f = 0.70;
    total_grip_cap_wheel = mu_max * (Fz_f_total(1) + Fz_r_total(1)) * Rw * 0.90;
    
    T_req_total_wheel = pedal(1) * total_grip_cap_wheel;
    T_req_front_wheel = T_req_total_wheel * bias_f;
    T_req_rear_wheel  = T_req_total_wheel * (1 - bias_f);
    
    T_f_fric = max(-mu_max * Fz_f_total(1) * Rw * 0.90, T_req_front_wheel);
    
    T_base_rr = max(-(T_grip_lim_rr_wheel - abs(T_delta_wheel_raw)), T_req_rear_wheel * weight_rr);
    T_base_rl = max(-(T_grip_lim_rl_wheel - abs(T_delta_wheel_raw)), T_req_rear_wheel * weight_rl);
    
    T_rr_ideal_wheel = T_base_rr + T_delta_wheel_raw;
    T_rl_ideal_wheel = T_base_rl - T_delta_wheel_raw;
    
    % Anti-Lock Braking (ABS)
    v_hub_fl = max(vx_curr(1) - (tw/2)*r_curr(1), 1.0);
    v_hub_fr = max(vx_curr(1) + (tw/2)*r_curr(1), 1.0);
    v_hub_rl = max(vx_curr(1) - (tw/2)*r_curr(1), 1.0);
    v_hub_rr = max(vx_curr(1) + (tw/2)*r_curr(1), 1.0);
    
    kappa_fl = (w_vec(1)*Rw - v_hub_fl) / v_hub_fl;
    kappa_fr = (w_vec(2)*Rw - v_hub_fr) / v_hub_fr;
    kappa_rl = (w_vec(3)*Rw - v_hub_rl) / v_hub_rl;
    kappa_rr = (w_vec(4)*Rw - v_hub_rr) / v_hub_rr;
    
    slip_limit_abs = -0.10;
    Kp_abs = 5000;
    
    worst_kappa_f = min(kappa_fl, kappa_fr);
    if worst_kappa_f < slip_limit_abs
        T_f_fric = min(0, T_f_fric - Kp_abs * (worst_kappa_f - slip_limit_abs));
    end
    
    if kappa_rl < slip_limit_abs
        T_rl_ideal_wheel = min(0, T_rl_ideal_wheel - Kp_abs * (kappa_rl - slip_limit_abs));
    end
    if kappa_rr < slip_limit_abs
        T_rr_ideal_wheel = min(0, T_rr_ideal_wheel - Kp_abs * (kappa_rr - slip_limit_abs));
    end
    
    T_rr_ideal = max(T_min_rr_motor, min(T_max_rr_motor, T_rr_ideal_wheel / G));
    T_rl_ideal = max(T_min_rl_motor, min(T_max_rl_motor, T_rl_ideal_wheel / G));
    
    T_rr_fric = max(-T_fric_max_per_wheel, min(0, T_rr_ideal_wheel - (T_rr_ideal * G)));
    T_rl_fric = max(-T_fric_max_per_wheel, min(0, T_rl_ideal_wheel - (T_rl_ideal * G)));
    
    if vx_curr(1) < 2.0
        T_f_fric = 0; T_rr_fric = 0; T_rl_fric = 0;
        T_rr_ideal = 0; T_rl_ideal = 0;
    end
end

T_rr_motor_raw = T_rr_ideal;
T_rl_motor_raw = T_rl_ideal;

end
